simulink model "mpcLKAsystem"  (R2022a)
settings: Solver=VariableStepAuto  StartTime=0.0  StopTime=15  RelTol=1e-3
values from neighbouring files (symbols this model uses):
  Cf = 19000    [Workspace.mat]
  Cr = 33000    [Workspace.mat]
  curvature = zeros(1,151)    [CurvatureToPath.m]    (also in Workspace.mat = [0 0 0 0 0 0 0 0 0 0 0 0 ... (151 elements, 1x151)])
  Iz = 2875    [Workspace.mat]
  lf = 1.2    [Workspace.mat]
  lr = 1.6    [Workspace.mat]
  m = 1575    [Workspace.mat]
  Ts = 0.1    [Workspace.mat]
  Vx = 15    [Workspace.mat]
libraries: mpcadaslib x1
settings Model: Creator=The MathWorks, Inc.  LastModifiedBy=Omkar
settings SolverCC: AlgebraicLoopSolver=TrustRegion
settings DataIOCC: ReturnWorkspaceOutputs=off
settings DebuggingCC: UnconnectedInputMsg=warning  UnconnectedOutputMsg=warning  UnconnectedLineMsg=warning  SFMachineParentedDataDiag=warning  ArithmeticOperatorsInVariantConditions=warning
settings SFSimCC: SimUseLocalCustomCode=off  CustomCodeUndefinedFunction=UseInterfaceOnly
settings RTWCC: RTWUseLocalCustomCode=off
settings CodeAppCC: StateflowObjectComments=on
settings SimscapeCC: SimscapeNormalizeSystem=off

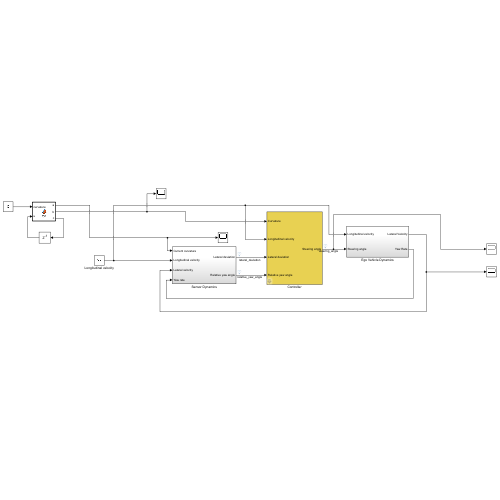
[thumbnail: Simulink's stored preview of the top-level diagram]
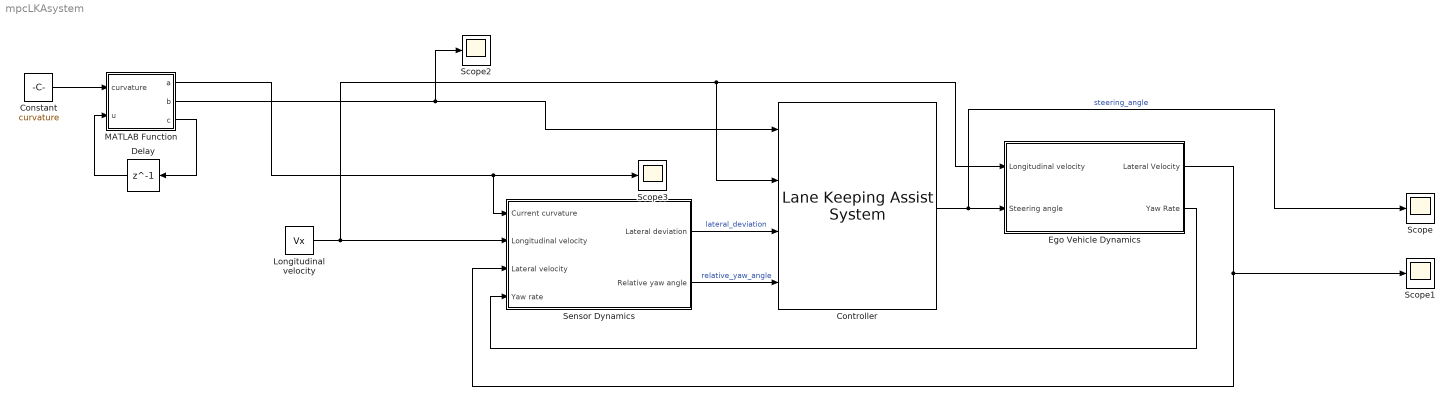
== system mpcLKAsystem ==
  Constant : Constant  Value=curvature  VectorParams1D=off
  Controller : mpcadaslib/Lane Keeping Assist System  ModelType=Use vehicle parameters  VehicleMass=1575  VehicleYawInertia=2875  LengthToFront=1.2  LengthToRear=1.6  FrontTireStiffness=19000  RearTireStiffness=33000  EgoModelMatrixA=[-4.4021 ,-12.4603;1.3913,-5.1868]  EgoModelMatrixB=[24.1270;15.8609]  EgoModelMatrixC=[1,0;0,1]  InitialLongVel=15  TransportLag=0  MinSteering=-0.26  umin_ext=off  MaxSteering=0.26  umax_ext=off  Ts=0.1  PredictionHorizon=10  ControllerBehavior=0.5  suboptimal=off  maxiter=10  datatypeopt=double  optmode=off  trackmode=off
      settings: SourceProductBaseCode=MP
  Delay : Delay  DelayLength=1  InitialCondition=1
  Ego Vehicle Dynamics : Subsystem
  Longitudinal velocity : Constant  Value=Vx  SampleTime=Ts
  MATLAB Function : MATLAB Function  TreatAsAtomicUnit=on
  Scope{,1..3} (4 alike) : Scope
  Sensor Dynamics : Subsystem
  wires:
  Ego Vehicle Dynamics/2(Yaw Rate) -> Sensor Dynamics/4(Yaw rate)
  Ego Vehicle Dynamics/1(Lateral Velocity) -> Sensor Dynamics/3(Lateral velocity), Scope1/1
  Sensor Dynamics/1(Lateral deviation) -> Controller/3  "lateral_deviation"
  Sensor Dynamics/2(Relative yaw angle) -> Controller/4  "relative_yaw_angle"
  Longitudinal velocity/1 -> Controller/2, Ego Vehicle Dynamics/1(Longitudinal velocity), Sensor Dynamics/2(Longitudinal velocity)
  MATLAB Function/2(b) -> Controller/1, Scope2/1
  Controller/1 -> Scope/1, Ego Vehicle Dynamics/2(Steering angle)  "steering_angle"
  MATLAB Function/1(a) -> Sensor Dynamics/1(Current curvature), Scope3/1
  Delay/1 -> MATLAB Function/2(u)
  MATLAB Function/3(c) -> Delay/1
  Constant/1 -> MATLAB Function/1(curvature)

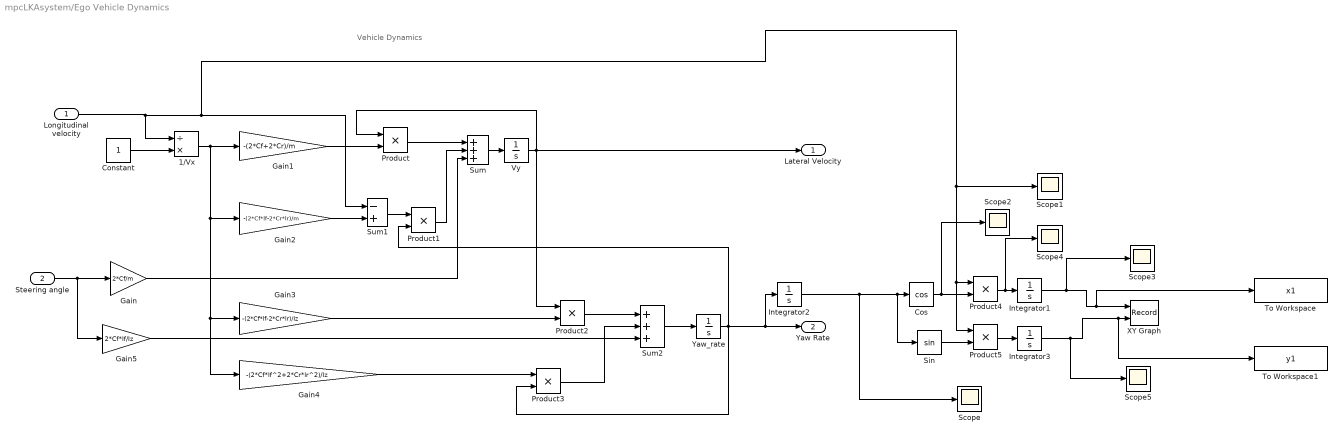
== system mpcLKAsystem/Ego Vehicle Dynamics ==
  note: Vehicle Dynamics
  Longitudinal velocity : Inport
  Steering angle : Inport  Port=2
  1/Vx : Product  Inputs=/*
  Constant : Constant
  Cos : Trigonometry  Operator=cos
  Gain : Gain  Gain=2*Cf/m
  Gain1 : Gain  Gain=-(2*Cf+2*Cr)/m
  Gain2 : Gain  Gain=-(2*Cf*lf-2*Cr*lr)/m
  Gain3 : Gain  Gain=-(2*Cf*lf-2*Cr*lr)/Iz
  Gain4 : Gain  Gain=-(2*Cf*lf^2+2*Cr*lr^2)/Iz
  Gain5 : Gain  Gain=2*Cf*lf/Iz
  Integrator1 : Integrator
  Integrator2 : Integrator
  Integrator3 : Integrator
  Product{,1..5} (6 alike) : Product
  Scope{,1..5} (6 alike) : Scope
  Sin : Trigonometry
  Sum : Sum  Inputs=+++
  Sum1 : Sum  Inputs=-+
  Sum2 : Sum  Inputs=+++
  To Workspace : ToWorkspace  VariableName=x1  SampleTime=0.1
  To Workspace1 : ToWorkspace  VariableName=y1  SampleTime=0.1
  Vy : Integrator
  XY Graph : Record  FileSettingsInternal="{\"entries\":[{\"content\":{\"excelSettings\":{\"content\":{},\"type\":\"Streamout.ExcelSettings\"}},\"type\":\"Streamout.FileSettingStorage\",\"uuid\":\"adf90c1e-e43d-4f8c-afac-554b430b79c0\"}],\"packageUris\":[\"http://schema.mathworks.com/mf0/streamout_blocks/R2020a\"],\"version\":\"1.0\"}"  Layout=[1 1]  SignalsInternal="{\"entries\":[{\"content\":{\"signals\":[{\"content\":{\"blockPath\":[\"mpcLKAsystem/Ego Vehicle Dynamics/XY Graph\"],\"channel\":[],\"dimensions\":[1],\"domain\":\"mpcLKAsystem/Ego Vehicle Dynamics/XY Graph\",\"lineColor\":\"#a2142f\",\"plots\":[1],\"port\":1,\"sid\":[\"\"],\"signalID\":2685,\"signalName\":\"Integrator1\"},\"type\":\"RecordBlkView.Signal\",\"uuid\":\"e010a4e8-004c-4329-88c9-80c03504fbf2\"},{\"content\":{\"blockPath\":[\"mpcLKAsystem/Ego Vehicle Dynamics/XY Graph\"],\"channel\":[],\"dimensions\":[1],\"domain\":\"mpcLKAsystem/Ego Vehicle Dynamics/XY Graph\",\"lineColor\":\"#139fff\",\"plots\":[1],\"port\":2,\"sid\":[\"\"],\"signalID\":2689,\"signalName\":\"Integrator3\"},\"type\":\"RecordBlkView.Signal\",\"uuid\":\"c715a48c-6d0d-4506-997e-ba917a2b7c49\"}]},\"type\":\"RecordBlkView.InputSignals\",\"uuid\":\"fd1e30aa-2cb2-430a-82d3-dfee0e3f582e\"}],\"packageUris\":[\"http://schema.mathworks.com/mf0/streamout_blocks/R2020a\"],\"version\":\"1.0\"}"  VisualizationBindings="{\"xyplotplugin\":{\"info\":[{\"series\":[{\"bindingParametersList\":[{\"parameter\":\"X-Axis\",\"signalID\":2685,\"signalName\":\"Integrator1\"},{\"parameter\":\"Y-Axis\",\"signalID\":2689,\"signalName\":\"Integrator3\"}],\"seriesID\":54735}],\"subplotID\":1}]}}"  CompatibilityTag=XY
  "Yaw_rate " : Integrator
  Lateral Velocity : Outport  VectorParamsAs1DForOutWhenUnconnected=off
  Yaw Rate : Outport  Port=2  VectorParamsAs1DForOutWhenUnconnected=off
  wires:
  Sum2/1 -> "Yaw_rate "/1
  Gain2/1 -> Sum1/2
  Gain4/1 -> Product3/1
  Constant/1 -> 1/Vx/2
  Gain3/1 -> Product2/2
  1/Vx/1 -> Gain4/1, Gain3/1, Gain2/1, Gain1/1
  Product2/1 -> Sum2/1
  Product3/1 -> Sum2/2
  Gain5/1 -> Sum2/3
  Sum1/1 -> Product1/1
  "Yaw_rate "/1 -> Product3/2, Integrator2/1, Yaw Rate/1, Product1/2
  Gain/1 -> Sum/3
  Steering angle/1 -> Gain/1, Gain5/1
  Gain1/1 -> Product/2
  Product/1 -> Sum/1
  Vy/1 -> Product/1, Lateral Velocity/1, Product2/1
  Sum/1 -> Vy/1
  Longitudinal velocity/1 -> Scope1/1, Product5/1, Product4/1, Sum1/1, 1/Vx/1
  Product1/1 -> Sum/2
  Integrator2/1 -> Scope/1, Sin/1, Cos/1
  Cos/1 -> Scope2/1, Product4/2
  Product4/1 -> Scope4/1, Integrator1/1
  Sin/1 -> Product5/2
  Product5/1 -> Integrator3/1
  Integrator3/1 -> Scope5/1, To Workspace1/1, XY Graph/2
  Integrator1/1 -> Scope3/1, To Workspace/1, XY Graph/1

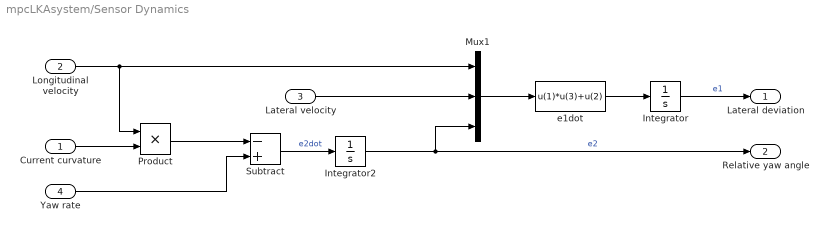
== system mpcLKAsystem/Sensor Dynamics ==
  Current curvature : Inport
  Longitudinal velocity : Inport  Port=2
  Lateral velocity : Inport  Port=3
  Yaw rate : Inport  Port=4
  Integrator : Integrator
  Integrator2 : Integrator
  Mux1 : Mux  Inputs=[1 1 1]
  Product : Product
  Subtract : Sum  Inputs=-+
  e1dot : Fcn  Expr=u(1)*u(3)+u(2)
  Lateral deviation : Outport  VectorParamsAs1DForOutWhenUnconnected=off
  Relative yaw angle : Outport  Port=2  VectorParamsAs1DForOutWhenUnconnected=off
  wires:
  Current curvature/1 -> Product/2
  Integrator2/1 -> Mux1/3, Relative yaw angle/1  "e2"
  Mux1/1 -> e1dot/1
  e1dot/1 -> Integrator/1
  Longitudinal velocity/1 -> Product/1, Mux1/1
  Lateral velocity/1 -> Mux1/2
  Integrator/1 -> Lateral deviation/1  "e1"
  Product/1 -> Subtract/1
  Yaw rate/1 -> Subtract/2
  Subtract/1 -> Integrator2/1  "e2dot"

== matlab function mpcLKAsystem/MATLAB Function ==
  data: curvature input; a output; b output; c output; u input
function [a, b, c] = fcn(curvature, u)
c=u;
d=u;
g=curvature;
a=g(c);
b=zeros(1,11);
for i=1:11
    if d<152
        b(i)=g(d);
    else
        b(i)=g(151)
    end
    d=1+d;
end

c=1+c;
end
